simulink model "Phil_VMP_DP_Combo_Task"  (R2013a)
settings: Solver=ode4  SolverMode=SingleTasking  StartTime=0.0  StopTime=inf  FixedStep=BKIN_STEP_TIME  RelTol=1e-3
StartFcn:
  |  warndlg('Dexterit-E models cannot run under simulation. Please compile your model and run it from within Dexterit-E.');set_param(bdroot,'SimulationCommand','stop')
model workspace (MAT data in the model file):
  col_x = 1
  col_y = 2
  RADIUS_VIS = 3
  COLOR_INIT = 4
  START_TARGET_COL = 1
  DELAY_POST_TRIAL_COL = 6
  MAX_REACH_TIME_COL = 4
  DELAY_COL = 5
  BKIN_STEP_TIME = 0.0005
  E_TRIAL_SUCCESS = 8
  SECOND_TARGET_COL = 3
  E_SECOND_TARGET_ON = 4
  WAIT_IN_HOME_COL = 2
  RADIUS_FUNC = 5
  E_SECOND_TARGET_REACHED = 5
  E_TRIAL_FAILURE = 7
  E_NEW_TRIAL = 3
  E_HOME_TARGET_REACHED = 2
  E_SHOW_HOME_TARGET = 6
  LOAD = 1
  TRIAL_TYPE_COL = 7
  RH_LOAD_COL = 8
  Cursor_Diameter_COL = 1
  SPEED_THRESHOLD_START = 2
  GOLDILOCKS = 6
  TOO_FAST = 8
  TOO_SLOW = 7
  LENGTH = 9
  WIDTH = 10
  ROTATION = 11
  SPEED_FEEDBACK_COL = 11
  GOLDILOCKS_COL = 12
  TOO_SLOW_COL = 13
  BASELINE_EEG_COL = 14
  BASELINE_DUR_COL = 15
  E_EEG_BASELINE = 1
  FORCE_CHANNEL_COL = 16
  WALL_WIDTH = 2
  CHANNEL_WIDTH = 3
  VISCOSITY = 4
  E_DEFINE_TRIAL_TYPE = 9
  CHANNEL_LOAD_COL = 17
  HAND_SPEED_THRESHOLD_COL = 18
  E_MOVEMENT_START = 10
  E_BASELINE_END = 11
  ROTATION_ANGLE_COL = 19
  VIS_VS_KIN_COL = 9
  DISTANCE_TO_HOME_COL = 10
  ROTATION_TYPE_COL = 20
  CONST_VISC_FORCE_COL = 21
  VISC_X = 5
  CURL_X = 6
  CURL_Y = 7
  VISC_Y = 8
undefined symbols (not defined in the file): Hand_Feedback, KINARM_DistanceFromTarget, KINARM_general, KINARM_HandInTarget, slselsubs
libraries: xpclib x6, KINARM_EP_loads x4, General x3, Video x3, xpcnilib x1
(part 2 of 3)

== system Phil_VMP_DP_Combo_Task/Create_MirrorTarget_Table ==
  note: The Goto block creates a tag that Simulink allows you to reference anywhere else in the Simulink model.
      | In this example, the goto tag is called "Mirror_Target_Table".  Please see the Simulink documentation for more
      | details on using Goto and From tags.
  Embedded MATLAB Mirror Target Table : MATLAB Function  TreatAsAtomicUnit=on
  Sho_X : Selector  NumberOfDimensions=2  InputPortWidth=3  IndexOptions=Index vector (dialog),Index vector (dialog)  Indices=[1:2],[4]  OutputSizes=1
  tag scope: Midline_Target_Table=global, Mirror_Target_Table=global
  wires:
  [Target_Table] -> Embedded MATLAB Mirror Target Table/2(Target_Table)
  [KINdata] -> Sho_X/1
  Embedded MATLAB Mirror Target Table/1(Mirror_Target_Table) -> [Mirror_Target_Table]
  Sho_X/1 -> Embedded MATLAB Mirror Target Table/1(shoulderXpos)
  Embedded MATLAB Mirror Target Table/2(Midline_Target_Table) -> [Midline_Target_Table]

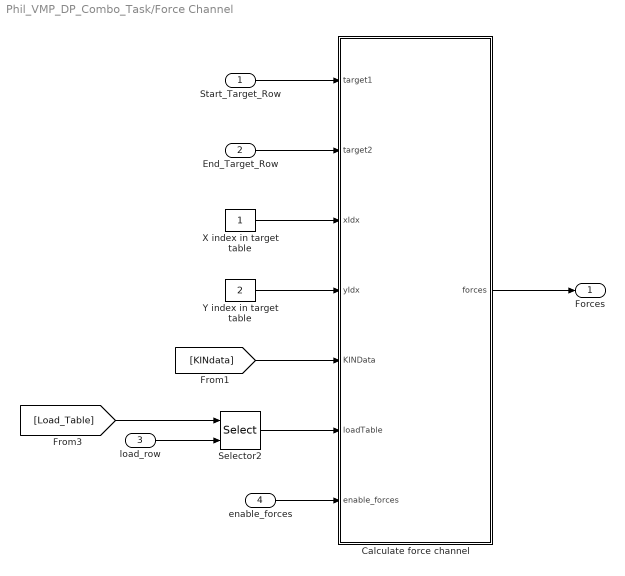
== system Phil_VMP_DP_Combo_Task/Force Channel ==
  Start_Target_Row : Inport
  End_Target_Row : Inport  Port=2
  load_row : Inport  Port=3
  enable_forces : Inport  Port=4
  Calculate force channel : MATLAB Function  TreatAsAtomicUnit=on
  Selector2 : Selector  NumberOfDimensions=2  InputPortWidth=3  IndexOptions=Index vector (port),Select all  Indices=1,-1  OutputSizes=slselsubs([(-2),(-2)],1),slselsubs([(-2),(-2)],2)
  X index in target table : Constant
  Y index in target table : Constant  Value=2
  Forces : Outport
  wires:
  [KINdata] -> Calculate force channel/5(KINData)
  X index in target table/1 -> Calculate force channel/3(xIdx)
  Y index in target table/1 -> Calculate force channel/4(yIdx)
  enable_forces/1 -> Calculate force channel/7(enable_forces)
  Calculate force channel/1(forces) -> Forces/1
  [Load_Table] -> Selector2/1
  load_row/1 -> Selector2/2
  Selector2/1 -> Calculate force channel/6(loadTable)
  Start_Target_Row/1 -> Calculate force channel/1(target1)
  End_Target_Row/1 -> Calculate force channel/2(target2)

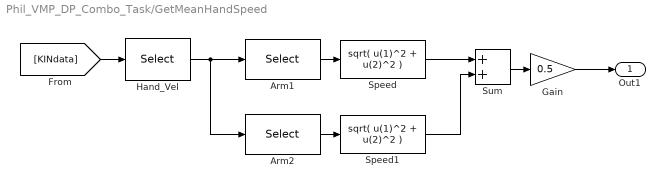
== system Phil_VMP_DP_Combo_Task/GetMeanHandSpeed ==
  Arm1 : Selector  NumberOfDimensions=2  InputPortWidth=3  IndexOptions=Index vector (dialog),Select all  Indices=1,-1  OutputSizes=1
  Arm2 : Selector  NumberOfDimensions=2  InputPortWidth=3  IndexOptions=Index vector (dialog),Select all  Indices=2,-1  OutputSizes=1
  Gain : Gain  Gain=0.5
  Hand_Vel : Selector  NumberOfDimensions=2  InputPortWidth=3  IndexOptions=Select all,Index vector (dialog)  Indices=-1,[25,26]  OutputSizes=1
  Speed : Fcn  Expr=sqrt( u(1)^2 + u(2)^2 )
  Speed1 : Fcn  Expr=sqrt( u(1)^2 + u(2)^2 )
  Sum : Sum
  Out1 : Outport
  wires:
  Arm2/1 -> Speed1/1
  Sum/1 -> Gain/1
  Hand_Vel/1 -> Arm1/1, Arm2/1
  Arm1/1 -> Speed/1
  [KINdata] -> Hand_Vel/1
  Speed/1 -> Sum/1
  Speed1/1 -> Sum/2
  Gain/1 -> Out1/1

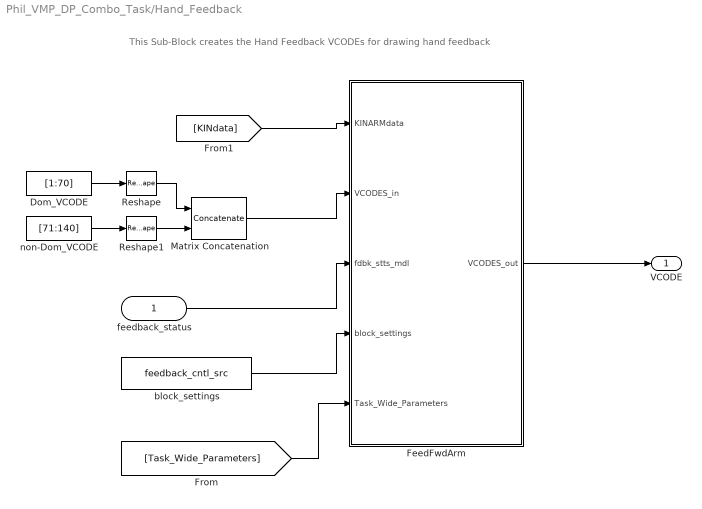
== system Phil_VMP_DP_Combo_Task/Hand_Feedback ==
  note: This Sub-Block creates the Hand Feedback VCODEs for drawing hand feedback
  feedback_status : Inport
  Dom_VCODE : Constant  Value=[1:70]
  FeedFwdArm : MATLAB Function  TreatAsAtomicUnit=on
  Matrix Concatenation : Concatenate  Mode=Multidimensional array
  Reshape : Reshape  OutputDimensionality=Row vector (2-D)
  Reshape1 : Reshape  OutputDimensionality=Row vector (2-D)
  block_settings : Constant  Value=feedback_cntl_src
  non-Dom_VCODE : Constant  Value=[71:140]
  VCODE : Outport
  wires:
  FeedFwdArm/1(VCODES_out) -> VCODE/1
  block_settings/1 -> FeedFwdArm/4(block_settings)
  Matrix Concatenation/1 -> FeedFwdArm/2(VCODES_in)
  [KINdata] -> FeedFwdArm/1(KINARMdata)
  Reshape1/1 -> Matrix Concatenation/2
  Reshape/1 -> Matrix Concatenation/1
  Dom_VCODE/1 -> Reshape/1
  non-Dom_VCODE/1 -> Reshape1/1
  feedback_status/1 -> FeedFwdArm/3(fdbk_stts_mdl)
  [Task_Wide_Parameters] -> FeedFwdArm/5(Task_Wide_Parameters)

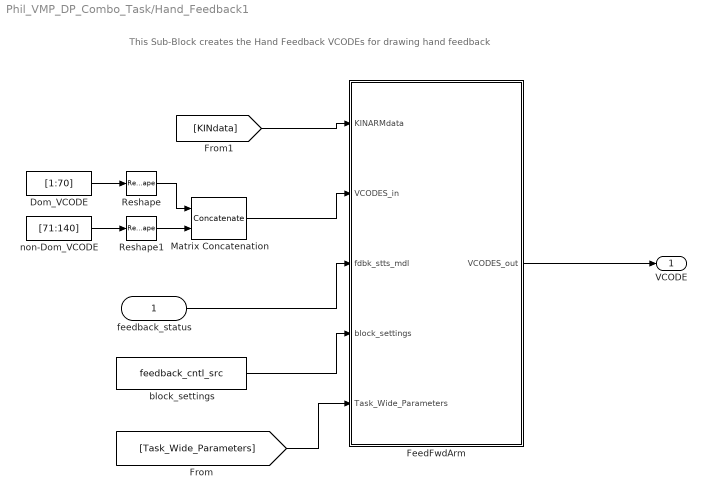
== system Phil_VMP_DP_Combo_Task/Hand_Feedback1 ==
  note: This Sub-Block creates the Hand Feedback VCODEs for drawing hand feedback
  feedback_status : Inport
  Dom_VCODE : Constant  Value=[1:70]
  FeedFwdArm : MATLAB Function  TreatAsAtomicUnit=on
  Matrix Concatenation : Concatenate  Mode=Multidimensional array
  Reshape : Reshape  OutputDimensionality=Row vector (2-D)
  Reshape1 : Reshape  OutputDimensionality=Row vector (2-D)
  block_settings : Constant  Value=feedback_cntl_src
  non-Dom_VCODE : Constant  Value=[71:140]
  VCODE : Outport
  wires:
  block_settings/1 -> FeedFwdArm/4(block_settings)
  Matrix Concatenation/1 -> FeedFwdArm/2(VCODES_in)
  [KINdata] -> FeedFwdArm/1(KINARMdata)
  Reshape1/1 -> Matrix Concatenation/2
  Reshape/1 -> Matrix Concatenation/1
  Dom_VCODE/1 -> Reshape/1
  non-Dom_VCODE/1 -> Reshape1/1
  feedback_status/1 -> FeedFwdArm/3(fdbk_stts_mdl)
  FeedFwdArm/1(VCODES_out) -> VCODE/1
  [Task_Wide_Parameters] -> FeedFwdArm/5(Task_Wide_Parameters)

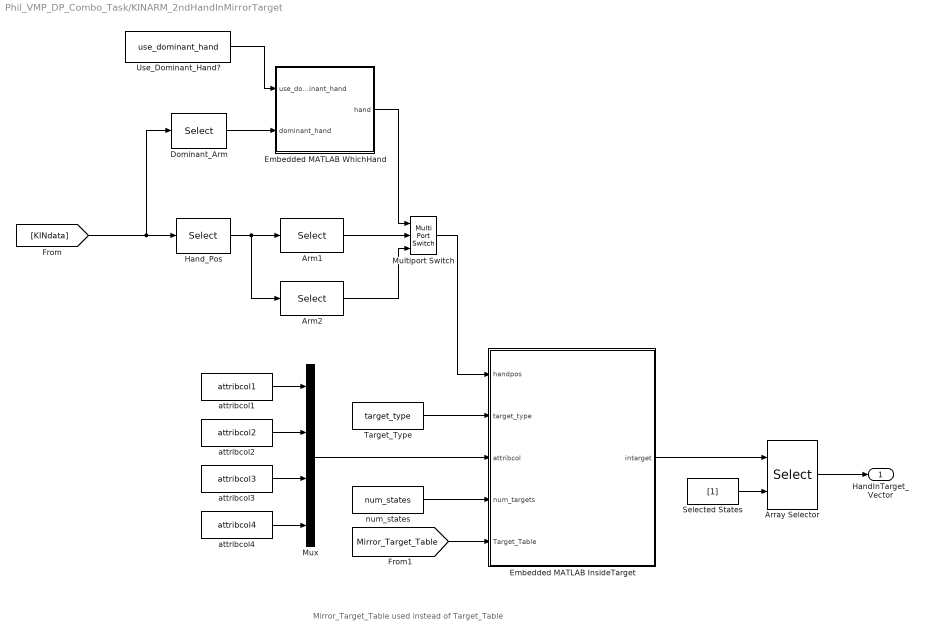
== system Phil_VMP_DP_Combo_Task/KINARM_2ndHandInMirrorTarget ==
  note: Mirror_Target_Table used instead of Target_Table
  Arm1 : Selector  NumberOfDimensions=2  InputPortWidth=3  IndexOptions=Index vector (dialog),Select all  Indices=1,-1  OutputSizes=slselsubs([(-2),(-2)],1),slselsubs([(-2),(-2)],2)
  Arm2 : Selector  NumberOfDimensions=2  InputPortWidth=3  IndexOptions=Index vector (dialog),Select all  Indices=2,-1  OutputSizes=slselsubs([(-2),(-2)],1),slselsubs([(-2),(-2)],2)
  Array Selector : Selector  NumberOfDimensions=2  InputPortWidth=3  IndexOptions=Select all,Index vector (port)  Indices=-1,1  OutputSizes=slselsubs([(-2),(-2)],1),slselsubs([(-2),(-2)],2)
  Dominant_Arm : Selector  NumberOfDimensions=2  InputPortWidth=3  IndexOptions=Index vector (dialog),Index vector (dialog)  Indices=[3],[1]  OutputSizes=slselsubs([(-2),(-2)],1),slselsubs([(-2),(-2)],2)
  Embedded MATLAB InsideTarget : MATLAB Function  TreatAsAtomicUnit=on
  Embedded MATLAB WhichHand : MATLAB Function  TreatAsAtomicUnit=on
  Hand_Pos : Selector  NumberOfDimensions=2  InputPortWidth=3  IndexOptions=Select all,Index vector (dialog)  Indices=-1,[23,24]  OutputSizes=slselsubs([(-2),(-2)],1),slselsubs([(-2),(-2)],2)
  Multiport Switch : MultiPortSwitch  Inputs=2
  Mux : Mux
  Selected States : Constant  Value=[1]
  Target_Type : Constant  Value=target_type
  Use_Dominant_Hand? : Constant  Value=use_dominant_hand
  attribcol1 : Constant  Value=attribcol1
  attribcol2 : Constant  Value=attribcol2
  attribcol3 : Constant  Value=attribcol3
  attribcol4 : Constant  Value=attribcol4
  num_states : Constant  Value=num_states
  HandInTarget_Vector : Outport
  wires:
  Selected States/1 -> Array Selector/2
  num_states/1 -> Embedded MATLAB InsideTarget/4(num_targets)
  Mux/1 -> Embedded MATLAB InsideTarget/3(attribcol)
  attribcol4/1 -> Mux/4
  attribcol3/1 -> Mux/3
  attribcol2/1 -> Mux/2
  attribcol1/1 -> Mux/1
  Use_Dominant_Hand?/1 -> Embedded MATLAB WhichHand/1(use_dominant_hand)
  Embedded MATLAB WhichHand/1(hand) -> Multiport Switch/1
  Target_Type/1 -> Embedded MATLAB InsideTarget/2(target_type)
  Array Selector/1 -> HandInTarget_Vector/1
  [Mirror_Target_Table] -> Embedded MATLAB InsideTarget/5(Target_Table)
  Embedded MATLAB InsideTarget/1(intarget) -> Array Selector/1
  Multiport Switch/1 -> Embedded MATLAB InsideTarget/1(handpos)
  Arm2/1 -> Multiport Switch/3
  Arm1/1 -> Multiport Switch/2
  Dominant_Arm/1 -> Embedded MATLAB WhichHand/2(dominant_hand)
  Hand_Pos/1 -> Arm2/1, Arm1/1
  [KINdata] -> Dominant_Arm/1, Hand_Pos/1

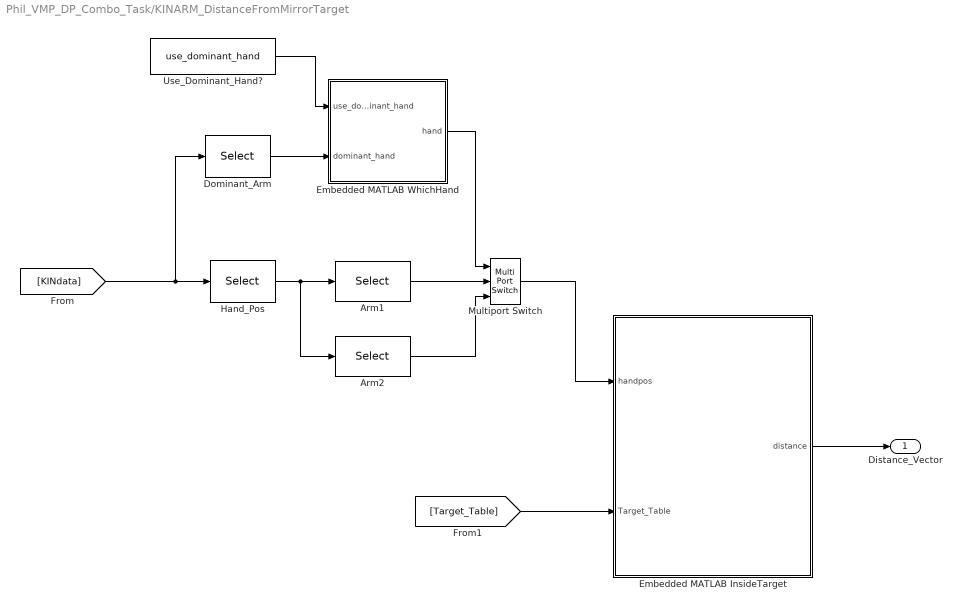
== system Phil_VMP_DP_Combo_Task/KINARM_DistanceFromMirrorTarget ==
  Arm1 : Selector  NumberOfDimensions=2  InputPortWidth=3  IndexOptions=Index vector (dialog),Select all  Indices=1,-1  OutputSizes=slselsubs([(-2),(-2)],1),slselsubs([(-2),(-2)],2)
  Arm2 : Selector  NumberOfDimensions=2  InputPortWidth=3  IndexOptions=Index vector (dialog),Select all  Indices=2,-1  OutputSizes=slselsubs([(-2),(-2)],1),slselsubs([(-2),(-2)],2)
  Dominant_Arm : Selector  NumberOfDimensions=2  InputPortWidth=3  IndexOptions=Index vector (dialog),Index vector (dialog)  Indices=[3],[1]  OutputSizes=slselsubs([(-2),(-2)],1),slselsubs([(-2),(-2)],2)
  Embedded MATLAB InsideTarget : MATLAB Function  TreatAsAtomicUnit=on
  Embedded MATLAB WhichHand : MATLAB Function  TreatAsAtomicUnit=on
  Hand_Pos : Selector  NumberOfDimensions=2  InputPortWidth=3  IndexOptions=Select all,Index vector (dialog)  Indices=-1,[23,24]  OutputSizes=slselsubs([(-2),(-2)],1),slselsubs([(-2),(-2)],2)
  Multiport Switch : MultiPortSwitch  Inputs=2
  Use_Dominant_Hand? : Constant  Value=use_dominant_hand
  Distance_Vector : Outport
  wires:
  Embedded MATLAB InsideTarget/1(distance) -> Distance_Vector/1
  Use_Dominant_Hand?/1 -> Embedded MATLAB WhichHand/1(use_dominant_hand)
  Embedded MATLAB WhichHand/1(hand) -> Multiport Switch/1
  [Target_Table] -> Embedded MATLAB InsideTarget/2(Target_Table)
  Multiport Switch/1 -> Embedded MATLAB InsideTarget/1(handpos)
  Arm2/1 -> Multiport Switch/3
  Arm1/1 -> Multiport Switch/2
  Dominant_Arm/1 -> Embedded MATLAB WhichHand/2(dominant_hand)
  Hand_Pos/1 -> Arm2/1, Arm1/1
  [KINdata] -> Dominant_Arm/1, Hand_Pos/1

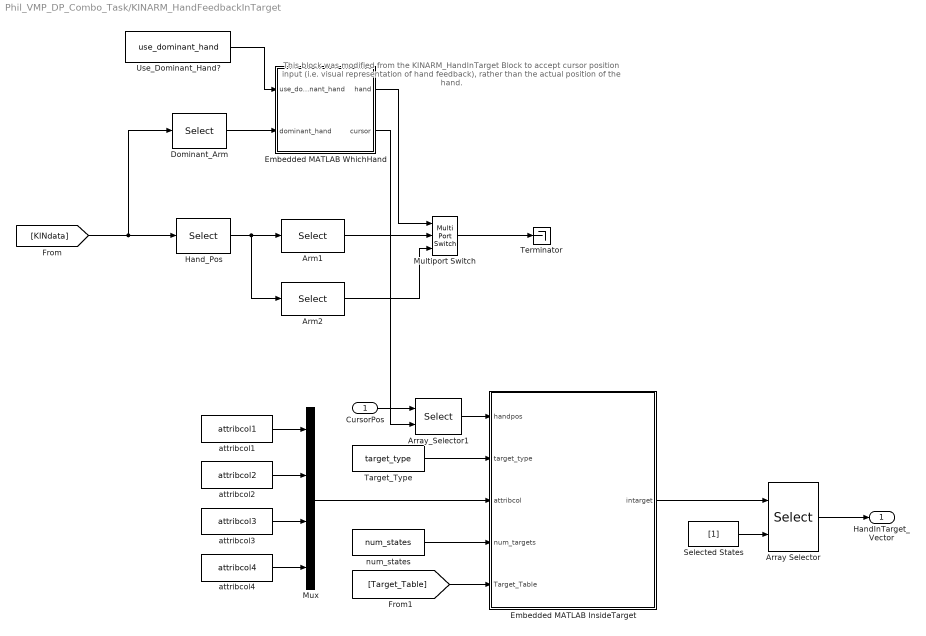
== system Phil_VMP_DP_Combo_Task/KINARM_HandFeedbackInTarget ==
  note: This block was modified from the KINARM_HandInTarget Block to accept cursor position input (i.e. visual
      | representation of hand feedback), rather than the actual position of the hand.
  CursorPos : Inport
  Arm1 : Selector  NumberOfDimensions=2  InputPortWidth=3  IndexOptions=Index vector (dialog),Select all  Indices=1,-1  OutputSizes=slselsubs([(-2),(-2)],1),slselsubs([(-2),(-2)],2)
  Arm2 : Selector  NumberOfDimensions=2  InputPortWidth=3  IndexOptions=Index vector (dialog),Select all  Indices=2,-1  OutputSizes=slselsubs([(-2),(-2)],1),slselsubs([(-2),(-2)],2)
  Array Selector : Selector  NumberOfDimensions=2  InputPortWidth=3  IndexOptions=Select all,Index vector (port)  Indices=-1,1  OutputSizes=slselsubs([(-2),(-2)],1),slselsubs([(-2),(-2)],2)
  Array_Selector1 : Selector  NumberOfDimensions=2  InputPortWidth=3  IndexOptions=Index vector (port),Select all  Indices=-1,1  OutputSizes=1
  Dominant_Arm : Selector  NumberOfDimensions=2  InputPortWidth=3  IndexOptions=Index vector (dialog),Index vector (dialog)  Indices=[3],[1]  OutputSizes=slselsubs([(-2),(-2)],1),slselsubs([(-2),(-2)],2)
  Embedded MATLAB InsideTarget : MATLAB Function  TreatAsAtomicUnit=on
  Embedded MATLAB WhichHand : MATLAB Function  TreatAsAtomicUnit=on
  Hand_Pos : Selector  NumberOfDimensions=2  InputPortWidth=3  IndexOptions=Select all,Index vector (dialog)  Indices=-1,[23,24]  OutputSizes=slselsubs([(-2),(-2)],1),slselsubs([(-2),(-2)],2)
  Multiport Switch : MultiPortSwitch  Inputs=2
  Mux : Mux
  Selected States : Constant  Value=[1]
  Target_Type : Constant  Value=target_type
  Terminator : Terminator
  Use_Dominant_Hand? : Constant  Value=use_dominant_hand
  attribcol1 : Constant  Value=attribcol1
  attribcol2 : Constant  Value=attribcol2
  attribcol3 : Constant  Value=attribcol3
  attribcol4 : Constant  Value=attribcol4
  num_states : Constant  Value=num_states
  HandInTarget_Vector : Outport
  wires:
  Selected States/1 -> Array Selector/2
  num_states/1 -> Embedded MATLAB InsideTarget/4(num_targets)
  Mux/1 -> Embedded MATLAB InsideTarget/3(attribcol)
  attribcol4/1 -> Mux/4
  attribcol3/1 -> Mux/3
  attribcol2/1 -> Mux/2
  attribcol1/1 -> Mux/1
  Use_Dominant_Hand?/1 -> Embedded MATLAB WhichHand/1(use_dominant_hand)
  Embedded MATLAB WhichHand/1(hand) -> Multiport Switch/1
  Target_Type/1 -> Embedded MATLAB InsideTarget/2(target_type)
  Array Selector/1 -> HandInTarget_Vector/1
  [Target_Table] -> Embedded MATLAB InsideTarget/5(Target_Table)
  Embedded MATLAB InsideTarget/1(intarget) -> Array Selector/1
  Multiport Switch/1 -> Terminator/1
  Arm2/1 -> Multiport Switch/3
  Arm1/1 -> Multiport Switch/2
  Dominant_Arm/1 -> Embedded MATLAB WhichHand/2(dominant_hand)
  Hand_Pos/1 -> Arm2/1, Arm1/1
  [KINdata] -> Dominant_Arm/1, Hand_Pos/1
  Array_Selector1/1 -> Embedded MATLAB InsideTarget/1(handpos)
  Embedded MATLAB WhichHand/2(cursor) -> Array_Selector1/2
  CursorPos/1 -> Array_Selector1/1

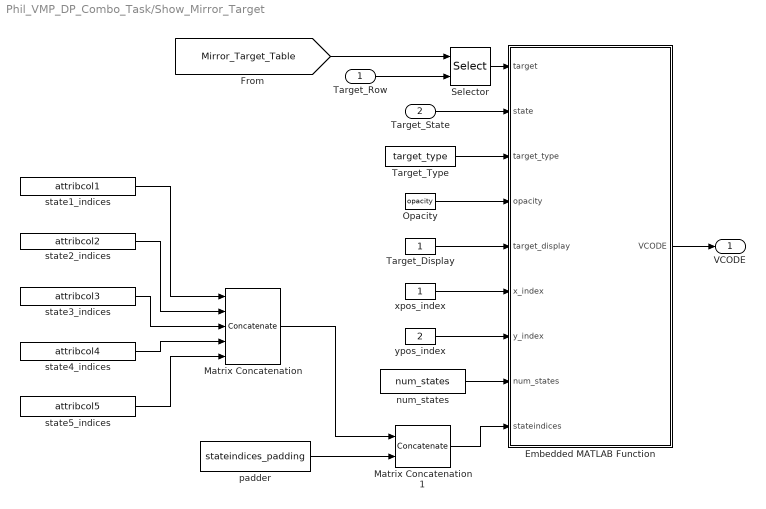
== system Phil_VMP_DP_Combo_Task/Show_Mirror_Target ==
  Target_Row : Inport
  Target_State : Inport  Port=2
  Embedded MATLAB Function : MATLAB Function  TreatAsAtomicUnit=on
  Matrix Concatenation : Concatenate  NumInputs=5  Mode=Multidimensional array
  Matrix Concatenation1 : Concatenate  Mode=Multidimensional array  ConcatenateDimension=2
  Opacity : Constant  Value=opacity
  Selector : Selector  NumberOfDimensions=2  InputPortWidth=3  IndexOptions=Index vector (port),Select all  Indices=1,-1  OutputSizes=slselsubs([(-2),(-2)],1),slselsubs([(-2),(-2)],2)
  Target_Display : Constant
  Target_Type : Constant  Value=target_type
  num_states : Constant  Value=num_states
  padder : Constant  Value=stateindices_padding
  state1_indices : Constant  Value=attribcol1  VectorParams1D=off
  state2_indices : Constant  Value=attribcol2  VectorParams1D=off
  state3_indices : Constant  Value=attribcol3  VectorParams1D=off
  state4_indices : Constant  Value=attribcol4  VectorParams1D=off
  state5_indices : Constant  Value=attribcol5  VectorParams1D=off
  xpos_index : Constant
  ypos_index : Constant  Value=2
  VCODE : Outport  PortDimensions=[1 70]
  wires:
  Target_Display/1 -> Embedded MATLAB Function/5(target_display)
  state2_indices/1 -> Matrix Concatenation/2
  state1_indices/1 -> Matrix Concatenation/1
  state5_indices/1 -> Matrix Concatenation/5
  state4_indices/1 -> Matrix Concatenation/4
  state3_indices/1 -> Matrix Concatenation/3
  Matrix Concatenation1/1 -> Embedded MATLAB Function/9(stateindices)
  padder/1 -> Matrix Concatenation1/2
  Matrix Concatenation/1 -> Matrix Concatenation1/1
  num_states/1 -> Embedded MATLAB Function/8(num_states)
  ypos_index/1 -> Embedded MATLAB Function/7(y_index)
  xpos_index/1 -> Embedded MATLAB Function/6(x_index)
  Target_Type/1 -> Embedded MATLAB Function/3(target_type)
  Embedded MATLAB Function/1(VCODE) -> VCODE/1
  Target_State/1 -> Embedded MATLAB Function/2(state)
  Selector/1 -> Embedded MATLAB Function/1(target)
  [Mirror_Target_Table] -> Selector/1
  Target_Row/1 -> Selector/2
  Opacity/1 -> Embedded MATLAB Function/4(opacity)

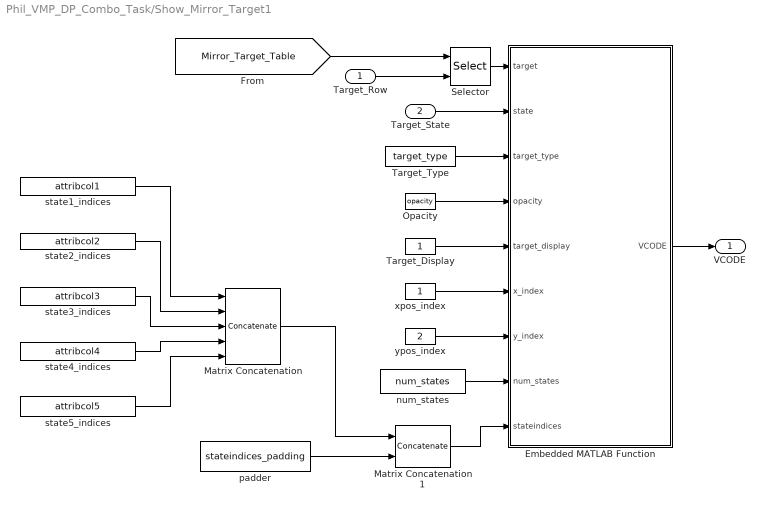
== system Phil_VMP_DP_Combo_Task/Show_Mirror_Target1 ==
  Target_Row : Inport
  Target_State : Inport  Port=2
  Embedded MATLAB Function : MATLAB Function  TreatAsAtomicUnit=on
  Matrix Concatenation : Concatenate  NumInputs=5  Mode=Multidimensional array
  Matrix Concatenation1 : Concatenate  Mode=Multidimensional array  ConcatenateDimension=2
  Opacity : Constant  Value=opacity
  Selector : Selector  NumberOfDimensions=2  InputPortWidth=3  IndexOptions=Index vector (port),Select all  Indices=1,-1  OutputSizes=slselsubs([(-2),(-2)],1),slselsubs([(-2),(-2)],2)
  Target_Display : Constant
  Target_Type : Constant  Value=target_type
  num_states : Constant  Value=num_states
  padder : Constant  Value=stateindices_padding
  state1_indices : Constant  Value=attribcol1  VectorParams1D=off
  state2_indices : Constant  Value=attribcol2  VectorParams1D=off
  state3_indices : Constant  Value=attribcol3  VectorParams1D=off
  state4_indices : Constant  Value=attribcol4  VectorParams1D=off
  state5_indices : Constant  Value=attribcol5  VectorParams1D=off
  xpos_index : Constant
  ypos_index : Constant  Value=2
  VCODE : Outport  PortDimensions=[1 70]
  wires:
  Target_Display/1 -> Embedded MATLAB Function/5(target_display)
  state2_indices/1 -> Matrix Concatenation/2
  state1_indices/1 -> Matrix Concatenation/1
  state5_indices/1 -> Matrix Concatenation/5
  state4_indices/1 -> Matrix Concatenation/4
  state3_indices/1 -> Matrix Concatenation/3
  Matrix Concatenation1/1 -> Embedded MATLAB Function/9(stateindices)
  padder/1 -> Matrix Concatenation1/2
  Matrix Concatenation/1 -> Matrix Concatenation1/1
  num_states/1 -> Embedded MATLAB Function/8(num_states)
  ypos_index/1 -> Embedded MATLAB Function/7(y_index)
  xpos_index/1 -> Embedded MATLAB Function/6(x_index)
  Target_Type/1 -> Embedded MATLAB Function/3(target_type)
  Embedded MATLAB Function/1(VCODE) -> VCODE/1
  Target_State/1 -> Embedded MATLAB Function/2(state)
  Selector/1 -> Embedded MATLAB Function/1(target)
  [Mirror_Target_Table] -> Selector/1
  Target_Row/1 -> Selector/2
  Opacity/1 -> Embedded MATLAB Function/4(opacity)

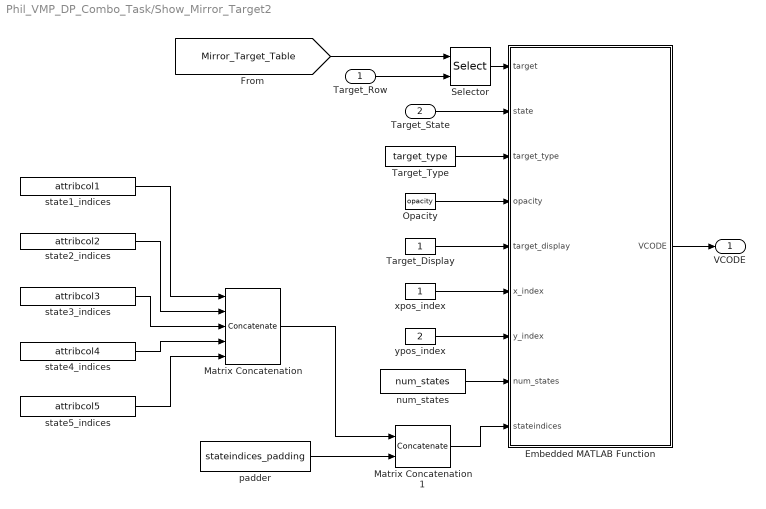
== system Phil_VMP_DP_Combo_Task/Show_Mirror_Target2 ==
  Target_Row : Inport
  Target_State : Inport  Port=2
  Embedded MATLAB Function : MATLAB Function  TreatAsAtomicUnit=on
  Matrix Concatenation : Concatenate  NumInputs=5  Mode=Multidimensional array
  Matrix Concatenation1 : Concatenate  Mode=Multidimensional array  ConcatenateDimension=2
  Opacity : Constant  Value=opacity
  Selector : Selector  NumberOfDimensions=2  InputPortWidth=3  IndexOptions=Index vector (port),Select all  Indices=1,-1  OutputSizes=slselsubs([(-2),(-2)],1),slselsubs([(-2),(-2)],2)
  Target_Display : Constant
  Target_Type : Constant  Value=target_type
  num_states : Constant  Value=num_states
  padder : Constant  Value=stateindices_padding
  state1_indices : Constant  Value=attribcol1  VectorParams1D=off
  state2_indices : Constant  Value=attribcol2  VectorParams1D=off
  state3_indices : Constant  Value=attribcol3  VectorParams1D=off
  state4_indices : Constant  Value=attribcol4  VectorParams1D=off
  state5_indices : Constant  Value=attribcol5  VectorParams1D=off
  xpos_index : Constant
  ypos_index : Constant  Value=2
  VCODE : Outport  PortDimensions=[1 70]
  wires:
  Target_Display/1 -> Embedded MATLAB Function/5(target_display)
  state2_indices/1 -> Matrix Concatenation/2
  state1_indices/1 -> Matrix Concatenation/1
  state5_indices/1 -> Matrix Concatenation/5
  state4_indices/1 -> Matrix Concatenation/4
  state3_indices/1 -> Matrix Concatenation/3
  Matrix Concatenation1/1 -> Embedded MATLAB Function/9(stateindices)
  padder/1 -> Matrix Concatenation1/2
  Matrix Concatenation/1 -> Matrix Concatenation1/1
  num_states/1 -> Embedded MATLAB Function/8(num_states)
  ypos_index/1 -> Embedded MATLAB Function/7(y_index)
  xpos_index/1 -> Embedded MATLAB Function/6(x_index)
  Target_Type/1 -> Embedded MATLAB Function/3(target_type)
  Embedded MATLAB Function/1(VCODE) -> VCODE/1
  Target_State/1 -> Embedded MATLAB Function/2(state)
  Selector/1 -> Embedded MATLAB Function/1(target)
  [Mirror_Target_Table] -> Selector/1
  Target_Row/1 -> Selector/2
  Opacity/1 -> Embedded MATLAB Function/4(opacity)

== system Phil_VMP_DP_Combo_Task/Visual vs. Kinesthetic Selector ==
  Trial_Protocol : Inport
  distance_from_target : Inport  Port=2
  reachingOut : Inport  Port=3
  MATLAB Function : MATLAB Function  TreatAsAtomicUnit=on
  feedback_status : Outport
  wires:
  Trial_Protocol/1 -> MATLAB Function/1(Trial_Protocol)
  MATLAB Function/1(y) -> feedback_status/1
  distance_from_target/1 -> MATLAB Function/2(distance_from_target)
  reachingOut/1 -> MATLAB Function/3(reachingOut)

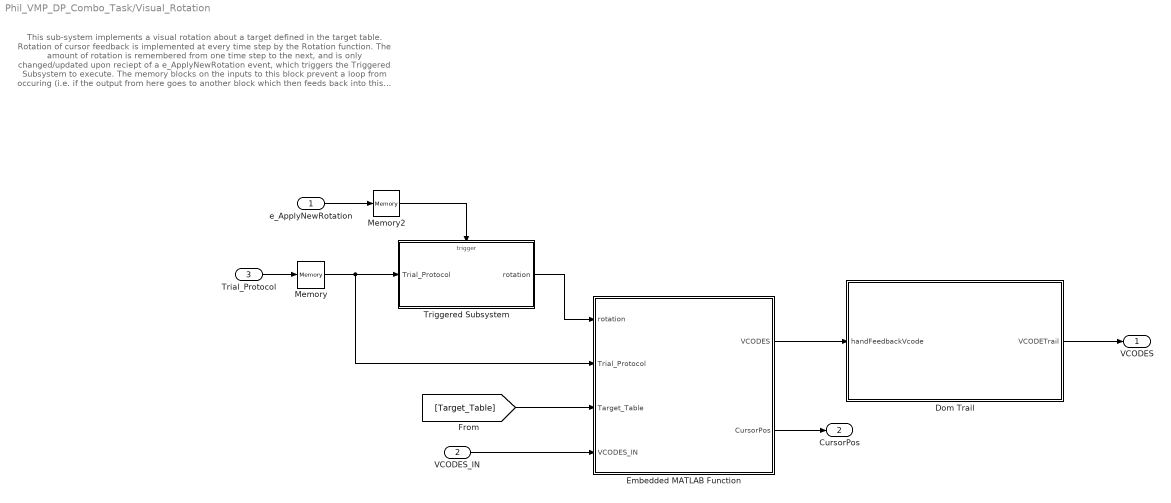
== system Phil_VMP_DP_Combo_Task/Visual_Rotation ==
  note: This sub-system implements a visual rotation about a target defined in the target table.
      |
      | Rotation of cursor feedback is implemented at every time step by the Rotation function.
      | The amount of rotation is remembered from one time step to the next, and is only changed/updated
      | upon reciept of a e_ApplyNewRotation event, which triggers the Triggered Subsystem to execute.
      |
      | The memory blocks on the inputs to this block prevent a loop from occuring (i.e. if the output from here goes to
      | another block which then feeds back into this block, which forms a loop, which needs to be broken by the Memory block).
  e_ApplyNewRotation : Inport
  VCODES_IN : Inport  Port=2
  Trial_Protocol : Inport  Port=3
  Dom Trail : MATLAB Function  TreatAsAtomicUnit=on
  Embedded MATLAB Function : MATLAB Function  TreatAsAtomicUnit=on
  Memory : Memory  InheritSampleTime=on
  Memory2 : Memory  InheritSampleTime=on
  Triggered Subsystem : Subsystem  TreatAsAtomicUnit=on
  VCODES : Outport
  CursorPos : Outport  Port=2
  wires:
  Trial_Protocol/1 -> Memory/1
  Embedded MATLAB Function/2(CursorPos) -> CursorPos/1
  Memory/1 -> Embedded MATLAB Function/2(Trial_Protocol), Triggered Subsystem/1(Trial_Protocol)
  e_ApplyNewRotation/1 -> Memory2/1
  Memory2/1 -> Triggered Subsystem/Trigger
  Triggered Subsystem/1(rotation) -> Embedded MATLAB Function/1(rotation)
  [Target_Table] -> Embedded MATLAB Function/3(Target_Table)
  VCODES_IN/1 -> Embedded MATLAB Function/4(VCODES_IN)
  Embedded MATLAB Function/1(VCODES) -> Dom Trail/1(handFeedbackVcode)
  Dom Trail/1(VCODETrail) -> VCODES/1

== system Phil_VMP_DP_Combo_Task/Visual_Rotation/Triggered Subsystem ==
  Trial_Protocol : Inport
  Trigger : TriggerPort  TriggerType=either
  Embedded MATLAB Function : MATLAB Function  TreatAsAtomicUnit=on
  rotation : Outport
  wires:
  Trial_Protocol/1 -> Embedded MATLAB Function/1(Trial_Protocol)
  Embedded MATLAB Function/1(rotation) -> rotation/1

== matlab function Phil_VMP_DP_Combo_Task/Visual_Rotation/Embedded MATLAB Function ==
  settings: fimath=|
      | fimath(...
      | 'RoundMode', 'floor',...
      | 'OverflowMode', 'wrap',...
      | 'ProductMode', 'KeepLSB', 'ProductWordLength', 32,...
      | 'SumMode', 'KeepLSB', 'SumWordLength', 32,...
      | 'CastBeforeSum', false)
  data: VCODES output; rotation input; Trial_Protocol input; Target_Table input; CursorPos output; VCODES_IN input
function [VCODES, CursorPos]  = Rotation(rotation, Trial_Protocol, Target_Table, VCODES_IN)
% This block supports an embeddable subset of the MATLAB language.
% See the help menu for details. 

%This block was modified by IEB, Sept 24, 2008
%It rotates the cursor position around a location specified as a target in the Trial_Protocol.

% VCODEs are length VCODE_LENGTH.
% All dimensions are units of (m).
% VCODE index definition: 1-5 as the same for all target types
% 1 - Target type
%		1=circle
%		2=ellipse
%       3=rectangle
%		4=line
%       5=triangle
%		6 and higher - not implemented yet
% 2 - status
%		0=off
%		1=on
% 3 - x position (m)
% 4 - y position (m)

% column in target table to find the target to rotation about
rotation_center_COL = 1;

rotation_center_target = Trial_Protocol(rotation_center_COL);
x_center = Target_Table(rotation_center_target, 1) * 0.01;		%convert to meters
y_center = Target_Table(rotation_center_target, 2) * 0.01;		%convert to meters

rotation = rotation*pi/180;		%convert desired rotation from degrees to radians

VCODES = VCODES_IN;
CursorPos = VCODES(1:2,3:4);
T = [x_center, y_center; x_center, y_center];                       %translation matrix
R = [cos(rotation) -sin(rotation); sin(rotation) cos(rotation)];	%rotation matrix

CursorPos = CursorPos - T;				%translate
CursorPos = (R*CursorPos')';			%rotate
CursorPos = CursorPos + T;				%re-translate

VCODES(1:2,3:4) = CursorPos;			%apply updated positions back into the VCODEs

== stateflow chart Phil_VMP_DP_Combo_Task/Trial Control ==
  state MainTrial
    state DefineTrialType/
      //1 = visual, 2 = kinesthetic, 3 = Baseline EEG
      trial_direction = Trial_Protocol[TRIAL_TYPE_COL];
      forces_enable = Trial_Protocol[FORCE_CHANNEL_COL];
      event_code = E_DEFINE_TRIAL_TYPE
      channel_row = Trial_Protocol[CHANNEL_LOAD_COL];
    state ShowSecondTarget/
      //Turn on second target and get participant moving to target
      targetA_row = Trial_Protocol[SECOND_TARGET_COL];
      targetA_state = 1;
      targetB_row = Trial_Protocol[SPEED_FEEDBACK_COL];
      targetB_state = 0;
      trial_abort = Trial_Protocol [MAX_REACH_TIME_COL];
      trial_type = Trial_Protocol[VIS_VS_KIN_COL];
      event_code = E_SECOND_TARGET_ON;
      event_code = E_HOME_TARGET_REACHED
      RH_load = Trial_Protocol[RH_LOAD_COL];
      reachingOut = 1;
      trigger1= 1;
    state StartMovementTimer/
      too_slow = Trial_Protocol[TOO_SLOW_COL];
      goldilocks = Trial_Protocol[GOLDILOCKS_COL];
      event_code = E_MOVEMENT_START;
      trigger2 = 1;
    state GOLDILOCKS_StayAtSecondTarget/
      // Log an event that target was reached and then wait for a specified time.
      //turn off load
      event_code = E_SECOND_TARGET_REACHED;
      tickCount = Trial_Protocol[DELAY_COL] ;
      targetB_state = 1;
      trigger3 =1;
    state TOO_SLOW_StayAtSecondTarget1/
      // Log an event that target was reached and then wait for a specified time.
      //turn off load
      event_code = E_SECOND_TARGET_REACHED;
      tickCount = Trial_Protocol[DELAY_COL] ;
      targetB_state = 2;
      trigger3=1;
    state TOO_FAST_StayAtSecondTarget2/
      // Log an event that target was reached and then wait for a specified time.
      //turn off load
      event_code = E_SECOND_TARGET_REACHED;
      tickCount = Trial_Protocol[DELAY_COL] ;
      targetB_state = 3;
      trigger3=1;
    state ReturnToHomeTarget/
      // Turn on home target and wait for a specified time or until the hand is in the target.
      targetA_row = Trial_Protocol[START_TARGET_COL];
      targetA_state = 1;
      event_code = E_SHOW_HOME_TARGET;
      reachingOut = 0;
      tickCount = Trial_Protocol[DELAY_POST_TRIAL_COL];
    state EndOfTrial/
      // Turn off the target, set the post-trial delay
      event_code = E_TRIAL_SUCCESS;
      event_code = E_HOME_TARGET_REACHED;
      targetB_state = 0;
    state TrialFail/
      tickCount = Trial_Protocol[DELAY_POST_TRIAL_COL];
      event_code = E_TRIAL_FAILURE;
    state BaselineEEG/
      // baseline EEG block
      targetA_row = Trial_Protocol[BASELINE_EEG_COL];
      targetA_state = 1;
      tickCount = Trial_Protocol[BASELINE_DUR_COL];
      event_code = E_EEG_BASELINE;
      trigger4 = 1;
    state EndBaseline/
      trigger5 = 1;
      event_code = E_BASELINE_END;
      targetA_state = 0;
    DefineTrialType -> BaselineEEG [order 1] : [trial_direction == 3]
    DefineTrialType -> ShowSecondTarget [order 2] : [after(tickCount, e_clk) && HandInTarget[targetA_row] == 1 && HandIn2ndTarget[targetA_row]==1]/
        | e_apply_new_rotation
    ShowSecondTarget -> TrialFail [order 1] : after(trial_abort,e_clk)
    ShowSecondTarget -> StartMovementTimer [order 2] : //After movement velocity is above threshold, start movement timer
        | [HandInTarget[Trial_Protocol[START_TARGET_COL]]==0 && HandIn2ndTarget[Trial_Protocol[START_TARGET_COL]]==0]
    StartMovementTimer -> GOLDILOCKS_StayAtSecondTarget [order 3] : [after(goldilocks, e_clk) && trial_type == 1 && HandInTarget[targetA_row] == 1 && MeanHandSpeed < Trial_Protocol[HAND_SPEED_THRESHOLD_COL]]
    StartMovementTimer -> GOLDILOCKS_StayAtSecondTarget [order 4] : // participant moves to target
        | // is the hand in the target?
        | [after(goldilocks, e_clk)  && trial_type == 0 && HandInTarget[targetA_row] == 1 && HandIn2ndTarget[targetA_row]==1 && MeanHandSpeed < Trial_Protocol[HAND_SPEED_THRESHOLD_COL]]
    StartMovementTimer -> TOO_SLOW_StayAtSecondTarget1 [order 1] : [after(too_slow, e_clk) && trial_type == 1 && HandInTarget[targetA_row] == 1 && MeanHandSpeed < Trial_Protocol[HAND_SPEED_THRESHOLD_COL]]
    StartMovementTimer -> TOO_SLOW_StayAtSecondTarget1 [order 2] : // participant moves to target
        | // is the hand in the target?
        | [after(too_slow, e_clk) && trial_type == 0 && HandInTarget[targetA_row] == 1 && HandIn2ndTarget[targetA_row]==1 && MeanHandSpeed < Trial_Protocol[HAND_SPEED_THRESHOLD_COL]]
    StartMovementTimer -> TOO_FAST_StayAtSecondTarget2 [order 5] : [trial_type == 1 && HandInTarget[targetA_row] == 1]
    StartMovementTimer -> TOO_FAST_StayAtSecondTarget2 [order 6] : // participant moves to target
        | // is the hand in the target?
        | // too fast does not require you to be at minimum speed to prevent participants from shooting out really fast and then adjusting to be in green
        | [trial_type == 0 && HandInTarget[targetA_row] == 1 && HandIn2ndTarget[targetA_row]==1]
    GOLDILOCKS_StayAtSecondTarget -> GOLDILOCKS_StayAtSecondTarget [order 1] : //are they still reaching?
        | [HandInTarget[targetA_row] == 0 || HandInTarget[targetA_row] == 0]
    TOO_FAST_StayAtSecondTarget2 -> TOO_FAST_StayAtSecondTarget2 [order 1] : //are they still reaching?
        | [HandInTarget[targetA_row] == 0 || HandInTarget[targetA_row] == 0]
    TOO_SLOW_StayAtSecondTarget1 -> TOO_SLOW_StayAtSecondTarget1 [order 1] : //are they still reaching?
        | [HandInTarget[targetA_row] == 0 || HandInTarget[targetA_row] == 0]
    GOLDILOCKS_StayAtSecondTarget -> ReturnToHomeTarget [order 2] : [trial_type == 1 && after(tickCount, e_clk) && HandInTarget[targetA_row] == 1]
    GOLDILOCKS_StayAtSecondTarget -> ReturnToHomeTarget [order 3] : // has a a specified period of
        | // time occured?
        | [trial_type ==0 && after(tickCount, e_clk) && HandInTarget[targetA_row]==1 && HandIn2ndTarget[targetA_row]==1]
    TOO_FAST_StayAtSecondTarget2 -> ReturnToHomeTarget [order 3] : [trial_type == 1 && after(tickCount, e_clk) && HandInTarget[targetA_row] == 1]
    TOO_FAST_StayAtSecondTarget2 -> ReturnToHomeTarget [order 2] : // has a a specified period of
        | // time occured?
        | [trial_type ==0 && after(tickCount, e_clk) && HandInTarget[targetA_row]==1 && HandIn2ndTarget[targetA_row]==1]
    TOO_SLOW_StayAtSecondTarget1 -> ReturnToHomeTarget [order 3] : [trial_type == 1 && after(tickCount, e_clk) && HandInTarget[targetA_row] == 1]
    TOO_SLOW_StayAtSecondTarget1 -> ReturnToHomeTarget [order 2] : // has a a specified period of
        | // time occured?
        | [trial_type ==0 && after(tickCount, e_clk) && HandInTarget[targetA_row]==1 && HandIn2ndTarget[targetA_row]==1]
    ReturnToHomeTarget -> EndOfTrial : [after(tickCount, e_clk) && HandInTarget[targetA_row]==1 && HandIn2ndTarget[targetA_row]==1]
    EndOfTrial -> EndOfTrial [order 1] : //are they still reaching?
        | [HandInTarget[targetA_row] == 0 || HandIn2ndTarget[targetA_row]== 0]
    BaselineEEG -> EndBaseline : after(tickCount, e_clk)
  state Initialiize/
    // If there was something to initialize
    // do it here
    targetA_row = Trial_Protocol[START_TARGET_COL];
    targetA_state = 1;
    event_code = E_SHOW_HOME_TARGET
    RH_load = Trial_Protocol[RH_LOAD_COL];
    tickCount = Trial_Protocol[WAIT_IN_HOME_COL];
    channel_row = Trial_Protocol[CHANNEL_LOAD_COL];
    const_visc_force = Trial_Protocol[CONST_VISC_FORCE_COL];
  state Inter_Trial_State/
    // Turn off target, reset the event code, and send the
    //e_Trial_End Stateflow event to indicate that the trial is over.
    e_Trial_End;
    event_code = E_NEW_TRIAL;
    targetA_row = Trial_Protocol[START_TARGET_COL];
    targetA_state = 1;
    targetB_state = 0;
    forces_enable = 0;
    tickCount = Trial_Protocol[WAIT_IN_HOME_COL]
    trigger1 = 0;
    trigger2 = 0;
    trigger3 = 0;
    trigger4 = 0;
    trigger5 = 0;
  (default) -> Initialiize
  Initialiize -> DefineTrialType
  Inter_Trial_State -> DefineTrialType : [HandInTarget[targetA_row] == 1 && HandIn2ndTarget[targetA_row]==1]/
  MainTrial -> Inter_Trial_State : e_ExitTrialNow/
      | tickCount = 1;
      | // e_ExitTrialNow event occurs if the
      | // Dex pause is pressed by the operator
  EndBaseline -> Inter_Trial_State : after(50, e_clk)
  TrialFail -> Inter_Trial_State : after(tickCount, e_clk)
  EndOfTrial -> Inter_Trial_State [order 2]
  data: random_number local double; event_code output uint16 [0..] =0; targetA_row output double [1..32]; targetA_state output double; tickCount local double; Trial_Protocol input double; HandInTarget input double; RH_load output double; trial_abort local double; HandIn2ndTarget input double; trial_type local double; reachingOut output double; targetB_row output double; targetB_state output double; too_slow local double; goldilocks local double; channel_row output double; forces_enable output double; MeanHandSpeed input double; trigger1 output double; trigger2 output double; trigger3 output double; trigger4 output double; trigger5 output double; const_visc_force output double; trial_direction local double
  data targetA_row settings: description=index of the row currently being used in the TargetTable
  events: e_clk input RISING_EDGE_EVENT; e_ExitTrialNow input EITHER_EDGE_EVENT; e_Trial_End output EITHER_EDGE_EVENT; e_apply_new_rotation output EITHER_EDGE_EVENT

== matlab function Phil_VMP_DP_Combo_Task/KINARM_2ndHandInMirrorTarget/Embedded MATLAB InsideTarget ==
  settings: fimath=|
      | fimath(...
      | 'RoundMode', 'floor',...
      | 'OverflowMode', 'wrap',...
      | 'ProductMode', 'KeepLSB', 'ProductWordLength', 32,...
      | 'SumMode', 'KeepLSB', 'SumWordLength', 32,...
      | 'CastBeforeSum', false)
  data: handpos input size=2; target_type input; attribcol input; num_targets input; intarget output; Target_Table input
function intarget = FIsInsideTarget(handpos, target_type, attribcol, num_targets, Target_Table)
% all dimensions in m, rad
% arguments:
% handpos: x,y positions of center of target
% attribcol: columns in target table specifying target attributes.  
% Specific to Target_Type
%	circle:
%	[X0,Y0,r...,rn] where:
%	X0,Y0 : centre of circle
%	r : logical radius of circle (i.e. radius used to determine 'in' or 'out' of target)
%	rn: logical radius of other targets (e.g. 2nd, 3rd) also specified in target row.
%   Up to 4 targets can be specified in a row
% ellipse:
%	[X0,Y0,a,b,t...,an, bn, tn] where:
%	X0,Y0 : centre of ellipse
%	a,b : major, minor radii of ellipse
%	t : rotation of ellipse in degrees
%	an,bn : major, minor radii of ellipse of other targets (e.g. 2nd, 3rd) also specified in target row
%	tn : rotation of ellipse in degrees of other targets (e.g. 2nd, 3rd) also specified in target row
%   Up to 4 targets can be specified in a row


target_col_x=1;
target_col_y=2;

x=handpos(1);
y=handpos(2);

intarget = zeros(size(Target_Table,1),4);

X0 = Target_Table(:,target_col_x)*0.01;			%Target Table sizes in cm in v1.4
Y0 = Target_Table(:,target_col_y)*0.01;			%Target Table sizes in cm in v1.4

deltax=x-X0;
deltay=y-Y0;

INT_MAX=2^32-1;

if target_type==1			%circle
	for target=1:num_targets
		r = Target_Table(:,attribcol(target))*0.01;			%Target Table sizes in cm in v1.4
		% simple euclidean distance
		distance2 = deltax.^2 + deltay.^2;					%distance2 is the square of the distance
	    intarget(:,target) = (distance2 <= r.^2);
	end
elseif target_type==2		%ellipse
	for target=1:num_targets
	    a = Target_Table(:,attribcol(target*3-2))*0.01;			%Target Table sizes in cm in v1.4
	    b = Target_Table(:,attribcol(target*3-1))*0.01;			%Target Table sizes in cm in v1.4	
	    t = Target_Table(:,attribcol(target*3))*(pi / 180.0);	%Target Table angles in degrees in v1.4
		sint=sin(t);
		cost=cos(t);
		xrotate=deltax.*cost+deltay.*sint;		%location of x point in ellipse's coordinate frame
		yrotate=-deltax.*sint+deltay.*cost;		%location of y point in ellipse's coordinate frame
		m=yrotate./xrotate;						%slope of line between the (x,y) to (x0,y0) in ellipse's coordinate frame
		y2sq=1./(1./(m.*a).^2+1./b.^2);			%y2sq is y2^2, where y2 is the intersection of the ellipse and the (x,y) to (x0,y0) line
	    intarget(:,target) = (yrotate.^2 <= y2sq);
    end
elseif target_type==3       %rectangle
    for target=1:num_targets
        w = Target_Table(:,attribcol(target*3-2))*0.01;  %width (sizes in cm in v1.4)
        h = Target_Table(:,attribcol(target*3-1))*0.01;  %height (sizes in cm in v1.4)
        
        if attribcol(target*3) > 0
            t = Target_Table(:,attribcol(target*3))*(pi / 180.0);  %angle (angles in degrees in v1.4)
        else
            t = zeros(size(Target_Table, 1), 1);
        end

        sint=sin(t);
        cost=cos(t);

        xrotate=deltax.*cost + deltay.*sint;   %location of x point in rectangle's coordinate frame
        yrotate=-deltax.*sint + deltay.*cost;  %location of y point in rectangle's coordinate frame

        intarget(:,target) = abs(xrotate) <= w/2 & abs(yrotate) <= h/2;
    end
elseif target_type==4       %line
    for target=1:num_targets
        % treat the line like a rectangle of height h and width w
        % determine height (stroke width) in the same fashion as in Show_Target
        if attribcol(target*3-2) == 0                     %0 column index means stroke width of 0
            h = zeros(size(Target_Table, 1), 1);
        elseif attribcol(target*3-2) < 0                  %-ve column index means stroke width of 1mm
            h = ones(size(Target_Table, 1), 1) .* 0.001;
        else
            h = Target_Table(:,attribcol(target*3-2)) * 0.01;  %target table contains width in cm
        end
        
        ex = Target_Table(:,attribcol(target*3-1))*0.01;  %endpoint in x relative to start point (cm)
        ey = Target_Table(:,attribcol(target*3))*0.01;    %endpoint in y relative to start point (cm)
        
        w = sqrt(ex.^2 + ey.^2);                          %width (cm)
        
        % determine the vector from the line's midpoint to the hand position
        handx = deltax - ex/2;
        handy = deltay - ey/2;
        
        t = atan2(ey, ex);                                %calculate angle of the line (rads)
        sint = sin(t);
        cost = cos(t);
        
        xrotate = handx.*cost + handy.*sint;   %location of x point in rectangle's coordinate frame
        yrotate = -handx.*sint + handy.*cost;  %location of y point in rectangle's coordinate frame
 
        intarget(:,target) = abs(xrotate) <= w/2 & abs(yrotate) <= h/2;
    end
elseif target_type==5  % triangle
    for target=1:num_targets
        w = Target_Table(:,attribcol(target*4-3))*0.01;         %length (sizes in cm in v1.4)
        
        % If a height column of 0 is specified, make the triangle equilateral. Otherwise, use the
        % values for height and peak offset from the target table.
        if attribcol(target*4-2) > 0
            h = Target_Table(:,attribcol(target*4-2))*0.01;  %height (sizes in cm in v1.4)
            p = Target_Table(:,attribcol(target*4-1))*0.01;  %peak offset (sizes in cm in v1.4)
        else
            h = w.*sin(pi/3.0);
            p = zeros(size(Target_Table, 1), 1);
        end
        
        if attribcol(target*4) > 0
            t = Target_Table(:,attribcol(target*4))*(pi / 180.0);  %angle (angles in degrees in v1.4)
        else
            t = zeros(size(Target_Table, 1), 1);
        end
        
        sint = sin(t);
        cost = cos(t);
        
        xrotate = deltax.*cost + deltay.*sint;   %location of x point in triangle's coordinate frame
        yrotate = -deltax.*sint + deltay.*cost;  %location of y point in triangle's coordinate frame
        
        % Begin to find centroid of triangle relative to the point on the base beneath the peak. "Left vertex" 
        % refers to the vertex at the left end of the base, and "right vertex" to the vertex at the right end.
        n = w./2.0 + p;  % distance along base from left vertex to peak
        m = w./2.0 - p;  % distance along base from peak to right vertex

        alpha = atan2(h, n);  % angle between base and line from left vertex to peak
        beta = atan2(h, m);   % angle between base and line from right vertex to peak
        
        length1 = sqrt(h.*h + n.*n) ./ 2.0;  % half length of line from left vertex to peak
        length2 = sqrt(h.*h + m.*m) ./ 2.0;  % half length of line from right vertex to peak

        % Determine slope of line from left vertex to midpoint of line from right vertex to peak.
        slope1 = ones(size(Target_Table, 1), 1) .* INT_MAX;
        
        for i=1:size(Target_Table, 1)
            if abs(w(i) - length2(i)*cos(beta(i))) > 0.0
                slope1(i) = length2(i)*sin(beta(i)) / (w(i) - length2(i)*cos(beta(i)));
            end
        end

        % Determine slope of line from right vertex to midpoint of line from left vertex to peak.
        slope2 = ones(size(Target_Table, 1), 1) .* INT_MAX;

        for i=1:size(Target_Table, 1)
            if abs(w(i) - length1(i)*cos(alpha(i))) > 0.0
                slope2(i) = -length1(i)*sin(alpha(i)) / (w(i) - length1(i)*cos(alpha(i)));
            end
        end

        % Calculate centroid position.
        centroid_x = -(m.*slope2 + n.*slope1) ./ (slope1 - slope2);
        centroid_y = slope1.*(centroid_x + n);

        % Test if the point is under the left side of the peak.
        is_under_left = false(size(Target_Table, 1), 1);

        for i=1:size(Target_Table, 1)
            if n(i) >= 0
                is_under_left(i) = (h(i) + (h(i)/n(i)) * (xrotate(i) + centroid_x(i))) >= (yrotate(i) + centroid_y(i));
            else
                is_under_left(i) = (h(i) + (h(i)/n(i)) * (xrotate(i) + centroid_x(i))) <= (yrotate(i) + centroid_y(i));
            end
        end
        
        % Test if the point is under the right side of the peak.
        is_under_right = false(size(Target_Table, 1), 1);

        for i=1:size(Target_Table, 1)
            if m(i) >= 0
                is_under_right(i) = (h(i) - (h(i)/m(i)) * (xrotate(i) + centroid_x(i))) >= (yrotate(i) + centroid_y(i));
            else
                is_under_right(i) = (h(i) - (h(i)/m(i)) * (xrotate(i) + centroid_x(i))) <= (yrotate(i) + centroid_y(i));
            end
        end
        
        intarget(:,target) = is_under_right & ...            %under right side of peak
                             is_under_left & ...             %under left side of peak
                             (yrotate + centroid_y) >= 0.0;  %above base
    end
end

== matlab function Phil_VMP_DP_Combo_Task/Show_Mirror_Target2/Embedded MATLAB Function ==
  settings: fimath=|
      | fimath(...
      | 'RoundMode', 'floor',...
      | 'OverflowMode', 'wrap',...
      | 'ProductMode', 'KeepLSB', 'ProductWordLength', 32,...
      | 'SumMode', 'KeepLSB', 'SumWordLength', 32,...
      | 'CastBeforeSum', false)
  data: target input; VCODE output; state input; target_type input; opacity input; target_display input; x_index input; y_index input; num_states input; stateindices input
function VCODE  = fcn(target, state, target_type, opacity, target_display, x_index, y_index, num_states, stateindices)

% VCODEs are length 70. All units in a VCODE should be SI, e.g. (m) and (rad). Elements in a VCODE are defined as follows:
%
% For all target types:
%  1: target type
%       1 - circle
%       2 - ellipse
%       3 - rectangle
%       4 - line
%       5 - triangle
%       11 - circle with label
%       12 - ellipse with label
%       13 - rectangle with label
%       14 - line with label
%       15 - triangle with label
%  2: target on/off status and target display (which display target will appear on)
%		0 - off
%		1 - on, appearing on both subject and operator displays
%       2 - on, appearing on subject display only
%       3 - on, appearing on operator display only
%  3: x position (m)
%  4: y position (m)
%  5: fill colour (RRGGBB) or texture index
%  6: stroke colour (RRGGBB) or texture index
%  7: stroke width
%  8: reserved for target background ID
%  9: opacity
%
% For circles:
%  10: radius (m)
%
% For ellipses:
%  10: major radius (m)
%  11: minor radius (m)
%  12: orientation of major axis (rad)
%
% For rectangles:
%  10: length (m)
%  11: height (m)
%  12: orientation (rad) (relative to x, y already shown)
%
% For lines:
%  10: endpoint x-axis coordinate relative to start point (m)
%  11: endpoint y-axis coordinate relative to start point (m)
%
% For triangles:
%  10: length (m)
%  11: height (m)
%  12: offset of peak from midpoint of length (m)
%  13: orientation (rad)
%
% For all labelled target types:
%  14: reserved
%  15-64: label characters (indexes in ISO 8859-1 character set)
%  65: label colour (0xRRGGBB), opacity is set by the vcode's opacity (9).
%  66: label height (m)
%  67: reserved
%  68: reserved
%  69: reserved
%  70: reserved

VCODE = zeros(1, 70);

% Set the target type.
VCODE(1) = target_type;

% Set the target on/off state. If the state input is 0, the target is off. Users of the VCODE should respect this
% as an indication that the rest of the VCODE will be uninitialized.
if (state <= 0) || (state > num_states)
	VCODE(2) = 0;  % target is off
	return;
else
	VCODE(2) = target_display;  % target is on; target displays as specified by block mask
end

% Set the target position.
VCODE(3) = target(x_index) * 0.01;  % x position (convert from (cm) in target table to (m))
VCODE(4) = target(y_index) * 0.01;  % y position (convert from (cm) in target table to (m))

% Set the fill colour. Fill colour currently comes from the GUI in RRRGGGBBB format.
if stateindices(state, 1) == 0
	VCODE(5) = -2^31;
elseif target(stateindices(state, 1)) < 0
    VCODE(5) = target(stateindices(state, 1));
else
	VCODE(5) = colourshift(target(stateindices(state, 1)));
end

% Set the stroke colour. Stroke colour currently comes from the GUI in RRRGGGBBB format.
if stateindices(state, 2) == 0
	VCODE(6) = -2^31;
elseif target(stateindices(state, 2)) < 0
    VCODE(6) = target(stateindices(state, 2));
else
	VCODE(6) = colourshift(target(stateindices(state, 2)));
end

% Set the stroke width. if target table index for stroke width is zero, then the stroke width is undefined
if stateindices(state, 3) == 0
	VCODE(7) = 0;                   % if stroke width column is 0, then stroke width is 0
elseif stateindices(state, 3) < 0
	VCODE(7) = 0.001;               % if stroke width column is -ve, then a 1mm default is chosen
else
	VCODE(7) = target(stateindices(state, 3)) * 0.01;  % if stroke width column is +ve, convert width from (cm) in target table to (m)
end

% Set the opacity value, clamping it to [0, 100].
if opacity <= 0
    VCODE(9) = 0.0;
elseif opacity >= 100
    VCODE(9) = 100.0;
else
    VCODE(9) = opacity;
end

% Set attributes specific to each target type.
if target_type == 1

    % Handle circle target:
	VCODE(10)=target(stateindices(state, 4)) * 0.01;  % radius (convert from (cm) in target table to (m))

elseif target_type == 2

    % Handle ellipse target:
	VCODE(10) = target(stateindices(state, 4)) * 0.01;  % major radius (convert from (cm) in target table to (m))
	VCODE(11) = target(stateindices(state, 5)) * 0.01;  % minor radius (convert from (cm) in target table to (m))

    if stateindices(state, 6) == 0
		VCODE(12) = 0;  % if orientation column is 0, set orientation to 0 rad
	else
		VCODE(12) = mod(target(stateindices(state, 6)), 360) * pi / 180.0;  % orientation (convert from (degrees) in target table to (rad))
    end

elseif target_type == 3

    % Handle rectangle target:
    VCODE(10) = target(stateindices(state, 4)) * 0.01;  % length (convert from (cm) in target table to (m))
    VCODE(11) = target(stateindices(state, 5)) * 0.01;  % height (convert from (cm) in target table to (m))

    if stateindices(state, 6) == 0
		VCODE(12) = 0;  % if orientation column is 0, set orientation to 0 rad
	else
		VCODE(12) = mod(target(stateindices(state, 6)), 360) * pi / 180.0;  % orientation (convert from (degrees) in target table to (rad))
    end
    
elseif target_type == 4

    % Handle line target:
    VCODE(10) = target(stateindices(state, 4)) * 0.01;  % line endpoint in x axis, relative to start (convert from (cm) in target table to (m))
    VCODE(11) = target(stateindices(state, 5)) * 0.01;  % line endpoint in y axis, relative to start (convert from (cm) in target table to (m))

elseif target_type == 5

    % Handle triangle target:
    VCODE(10) = target(stateindices(state, 4)) * 0.01;  % length (convert from (cm) in target table to (m))

    % If the height column is set to 0 then the triangle is automatically made equilateral, with the base length used as length
    % for all sides. If the height column is non-zero, separate values for height and peak offset are taken from the target table.
    if stateindices(state, 5) == 0
        VCODE(11) = sin(pi / 3.0) * VCODE(10);  % height for equilateral triangle
        VCODE(12) = 0;                          % peak offset for equilateral triangle
    else
        VCODE(11) = target(stateindices(state, 5)) * 0.01;  % height (convert from (cm) in target table to (m))
        VCODE(12) = target(stateindices(state, 6)) * 0.01;  % peak offset (convert from (cm) in target table to (m))
    end

    if stateindices(state, 7) == 0
        VCODE(13) = 0;  % if orientation column is 0, set orientation to 0 rad
    else
        VCODE(13) = mod(target(stateindices(state, 7)), 360) * pi / 180.0;  % orientation (convert from (degrees) in target table to (rad))
    end
end


% The colourshift function converts an "RRRGGGBBB" colour value to RRGBB (as an uint32).
function RRGGBBAA = colourshift(RRRGGGBBB)

blue = cast(mod(RRRGGGBBB, 1000), 'uint32');
green = cast(mod(RRRGGGBBB - blue, 1000000) / 1000, 'uint32');
red = cast((RRRGGGBBB - (green * 1000) - blue) / 1000000, 'uint32');

RRGGBBAA = bitshift(red, 16) + bitshift(green, 8) + blue;
